simulink model "gnc"  (R2025b)
settings: Solver=ode2  StartTime=0.0  StopTime=inf  FixedStep=1/100  RelTol=1e-3
PreLoadFcn:
  | gnc_PreLoadFcn
undefined symbols (not defined in the file or in its folder): DiscIntNeverNeededParam, dspblkCoreblockFVToolHelper, gcbh
libraries: simulink_extras x7, simulink x5, eeGeneralControl x5
(part 3 of 4)

== system gnc/Subsystem2/Actuator_Model/Actuator Model ==
  note: Discrete time actuator
      | dynamics transfer function
      | modelled as PT1 in
      | continuous time (tau = 0.05,
      | ts = 100Hz).
      | See filter_design.m for
      | more details.
  note: Actuator model output units need to
      | match increment units of control law.
      | Therefore, controller output must be
      | retransformed to corresponding unit.
  note: Current control surface
      | deflection in rad, thrust
      | lever in [0,1].
  note: Current actuator signal in %
      | Thrust [-1, 1]
      | Aileron [-1, 1]
      | Elevator [-1, 1]
      | Rudder [-1, 1]
  note: Scale actuator
      | signal from
      | % to rad
  note: Limit between
      | [-1,1]
  note: Limit
      | between
      | [0,1]
  note: Discrete time thrust
      | dynamics transfer function
      | modelled as PT1 in
      | continuous time (tau = 0.15,
      | ts = 100Hz).
      | See filter_design.m for
      | more details.
  note: Aileron		[-1, 1]
      | Elevator		[-1, 1]
      | Rudder		[-1, 1]
      | Thrust		[0, 1]
  note: Scale thrust signal
  RC_controls : Inport
  Safety_Switch : Inport  Port=2
  AP_controls : Inport  Port=3  OutDataTypeStr=Bus: main_ctrl_axes_bus
  act_lims : Inport  Port=4
  Bus Selector : BusSelector  OutputSignals=aileron,elevator,rudder,thrust
  Data Type Conversion1 : DataTypeConversion  OutDataTypeStr=single  SaturateOnIntegerOverflow=off  RndMeth=Floor
  Demux : Demux
  MATLAB Function1 : MATLAB Function  TreatAsAtomicUnit=on
  Mux : Mux  Inputs=3
  Mux1 : Mux  Inputs=2
  Mux4 : Mux
  Scope : Scope  NumInputPorts=4
  Scope1 : Scope  NumInputPorts=4
      settings: ActiveDisplayYMinimum=-0.125  ActiveDisplayYMaximum=1.125
  Scope2 : Scope
      settings: ActiveDisplayYMinimum=-1  ActiveDisplayYMaximum=1  DataLoggingVariableName=ScopeData8
  Switch1 : Switch  Criteria=u2 > Threshold  SaturateOnIntegerOverflow=off  InputSameDT=off
  act_alg : DiscreteTransferFcn  Numerator=[0.0909 0.0909]  Denominator=[1 -0.8182]
  act_alg2 : DiscreteTransferFcn  LoadFcn=dspblkCoreblockFVToolHelper(gcbh,'load');  Numerator=[0.0323 0.0323]  Denominator=[1 -0.9355]
      settings: CopyFcn=dspblkCoreblockFVToolHelper(gcbh,'copy');  DeleteFcn=dspblkCoreblockFVToolHelper(gcbh,'close');  ModelCloseFcn=dspblkCoreblockFVToolHelper(gcbh,'close');  PreSaveFcn=dspblkCoreblockFVToolHelper(gcbh,'presave');  PostSaveFcn=dspblkCoreblockFVToolHelper(gcbh,'postsave');  CloseFcn=dspblkCoreblockFVToolHelper(gcbh,'close');
  cmd2deg : MATLAB Function  TreatAsAtomicUnit=on
  limit control output : MATLAB Function  TreatAsAtomicUnit=on
  limit control output3 : MATLAB Function  TreatAsAtomicUnit=on
  Delayed : Outport
  wires:
  act_alg2/1 -> Scope1/1, Mux1/2
  limit control output3/1(y) -> Scope1/2, act_alg2/1, Scope1/3
  act_lims/1 -> cmd2deg/1(act_limits)
  Mux1/1 -> Data Type Conversion1/1
  act_alg/1 -> Scope/4, Mux1/1
  Demux/3 -> Mux/3
  Demux/1 -> Mux/1
  Demux/2 -> Mux/2
  AP_controls/1 -> Bus Selector/1
  Data Type Conversion1/1 -> Delayed/1
  Mux4/1 -> MATLAB Function1/1(in), Scope2/1
  Mux/1 -> Scope/1, limit control output/1(u)
  cmd2deg/1(y) -> Scope/3, act_alg/1
  limit control output/1(y) -> Scope/2, cmd2deg/2(u)
  MATLAB Function1/1(out) -> Switch1/3
  Bus Selector/4 -> Mux4/4  "<thrust>"
  Demux/4 -> Scope1/4, limit control output3/1(u)
  RC_controls/1 -> Switch1/1
  Safety_Switch/1 -> Switch1/2
  Switch1/1 -> Demux/1
  Bus Selector/1 -> Mux4/1  "<aileron>"
  Bus Selector/2 -> Mux4/2  "<elevator>"
  Bus Selector/3 -> Mux4/3  "<rudder>"

== system gnc/Subsystem2/Actuator_Model/Subsystem1 ==
  note: Input from Gram RC:
      | 1 Thrust
      | 2 Aileron
      | 3 Elevator
      | 4 Rudder
      | 5 Tail surface right
      | 6 Tail surface left
      | 7 Mode switch
      | 8 Arming
      | 9 Safety
  note: (1) test_controls
      | (2) steady_state
      | (3) wp_tracking
  note: Signal Limits:
      | Aileron		[-1, 1]
      | Elevator		[-1, 1]
      | Rudder		[-1, 1]
      | Thrust		[0, 1]
  note: [ Aileron	  ]
      | [ Elevator ]
      | [ Rudder	  ]
      | [ Thrust	  ]
  RC_channels : Inport  OutDataTypeStr=Bus: rc_channels_bus
  Bus Selector1 : BusSelector  OutputSignals=channels
  Demux1 : Demux  Outputs=6
  MATLAB Function : MATLAB Function  TreatAsAtomicUnit=on
  Mux : Mux
  Scope : Scope  NumInputPorts=2
      settings: ActiveDisplayYMinimum=-1.5  ActiveDisplayYMaximum=3.5  DataLoggingVariableName=ScopeData3
  Scope1 : Scope
      settings: ActiveDisplayYMinimum=-1.5  ActiveDisplayYMaximum=3.5  DataLoggingVariableName=ScopeData7
  Selector : Selector  InputPortWidth=18  IndexOptions=Index vector (dialog)  Indices=[2 3 4 1 7 9]  OutputSizes=1
  rc_mode : Outport  OutDataTypeStr=uint8
  RC_controls : Outport  Port=2
  Safety_Switch : Outport  Port=3
  wires:
  Demux1/3 -> Mux/3
  Demux1/1 -> Mux/1
  Demux1/2 -> Mux/2
  MATLAB Function/1(y) -> Scope/1, rc_mode/1
  Selector/1 -> Demux1/1
  Mux/1 -> RC_controls/1
  Demux1/5 -> MATLAB Function/1(u), Scope/2
  RC_channels/1 -> Bus Selector1/1
  Demux1/6 -> Safety_Switch/1, Scope1/1
  Demux1/4 -> Mux/4
  Bus Selector1/1 -> Selector/1  "<channels>"

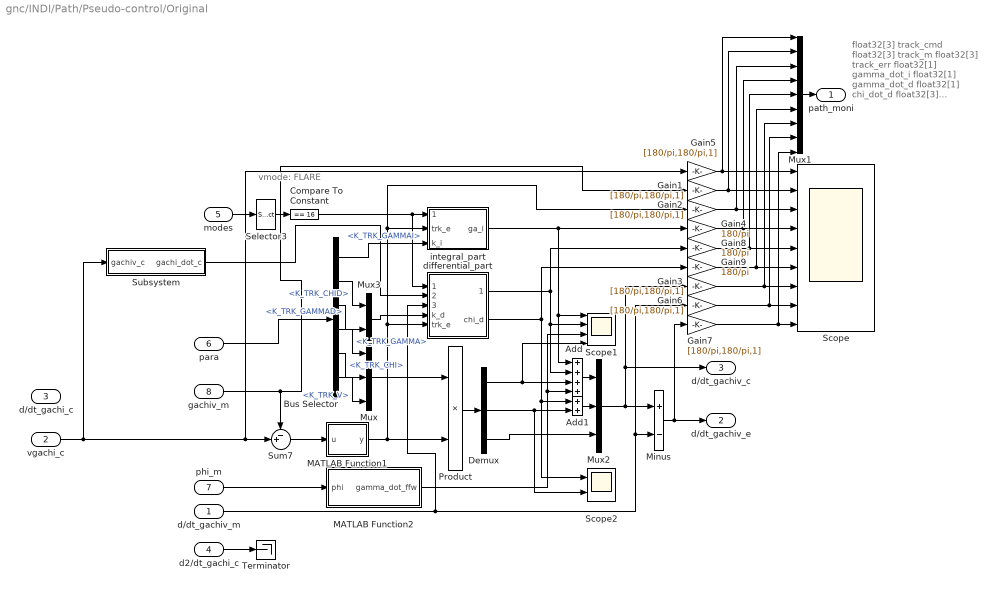
== system gnc/INDI/Path/Pseudo-control/Original ==
  note: float32[3] track_cmd
      | float32[3] track_m
      | float32[3] track_err
      | float32[1] gamma_dot_i
      | float32[1] gamma_dot_d
      | float32[1] chi_dot_d
      | float32[3] track_dot_cmd
      | float32[3] track_dot_m
      | float32[3] track_dot_err
  note: vmode: FLARE
  d/dt_gachiv_m : Inport  PortDimensions=3
  vgachi_c : Inport  Port=2
  d/dt_gachi_c : Inport  Port=3
  d2/dt_gachi_c : Inport  Port=4
  modes : Inport  Port=5  PortDimensions=4
  para : Inport  Port=6  OutDataTypeStr=Bus: gnc_parameterBus
  phi_m : Inport  Port=7
  gachiv_m : Inport  Port=8  PortDimensions=3
  Add : Sum  Inputs=++++
  Add1 : Sum
  Bus Selector : BusSelector  OutputSignals=indi.K_TRK_GAMMAI,indi.K_TRK_CHID,indi.K_TRK_GAMMAD,indi.K_TRK_GAMMA,indi.K_TRK_CHI,indi.K_TRK_V
  Compare To Constant : simulink/Logic and Bit Operations/Compare To Constant  relop===  const=16  OutDataTypeStr=boolean
  Demux : Demux  Outputs=3
  Gain{1..3,5..7} (6 alike) : Gain  Gain=[180/pi,180/pi,1]
  Gain4 : Gain  Gain=180/pi
  Gain8 : Gain  Gain=180/pi
  Gain9 : Gain  Gain=180/pi
  MATLAB Function1 : MATLAB Function  TreatAsAtomicUnit=on
  MATLAB Function2 : MATLAB Function  TreatAsAtomicUnit=on
  Minus : Sum  Inputs=+-
  Mux : Mux  Inputs=3
  Mux1 : Mux  Inputs=9
  Mux2 : Mux  Inputs=3
  Mux3 : Mux  Inputs=2
  Product : Product
  Scope : Scope  NumInputPorts=9
      settings: ActiveDisplayYMinimum=-85.31239  ActiveDisplayYMaximum=124.63703
  Scope1 : Scope  NumInputPorts=4
      settings: ActiveDisplayYMinimum=-1  ActiveDisplayYMaximum=1  DataLoggingVariableName=ScopeData2
  Scope2 : Scope  NumInputPorts=2
      settings: ActiveDisplayYMinimum=-1  ActiveDisplayYMaximum=1  DataLoggingVariableName=ScopeData2
  Selector3 : Selector  InputPortWidth=4  IndexOptions=Index vector (dialog)  Indices=1  OutputSizes=1
  Subsystem : Subsystem
  Sum7 : Sum  Inputs=-+|
  Terminator : Terminator
  differential_part : Subsystem
  integral_part : Subsystem
  path_moni : Outport
  d/dt_gachiv_e : Outport  Port=2  OutDataTypeStr=single  PortDimensions=3
  d/dt_gachiv_c : Outport  Port=3  OutDataTypeStr=single  PortDimensions=3
  wires:
  Gain6/1 -> Mux1/8, Scope/8
  vgachi_c/1 -> Subsystem/1(gachiv_c), Gain5/1, Sum7/2
  Minus/1 -> d/dt_gachiv_e/1, Gain7/1
  Gain4/1 -> Mux1/4, Scope/4
  Subsystem/1(gachi_dot_c) -> differential_part/2(gachi_dot_c)
  Gain9/1 -> Mux1/6, Scope/6
  Demux/1 -> Scope1/4, Add/3
  phi_m/1 -> MATLAB Function2/1(phi)
  Product/1 -> Demux/1
  Add1/1 -> Mux2/2
  Mux3/1 -> differential_part/4(k_d)
  Gain5/1 -> Mux1/1, Scope/1
  Gain7/1 -> Mux1/9, Scope/9
  Bus Selector/2 -> Mux3/1  "<K_TRK_CHID>"
  Sum7/1 -> MATLAB Function1/1(u)
  Compare To Constant/1 -> differential_part/1(flare_trig), integral_part/1(flare_trig)
  d/dt_gachiv_m/1 -> differential_part/3(gachiv_dot_m), Gain6/1, Minus/2
  Demux/3 -> Mux2/3
  Mux1/1 -> path_moni/1
  MATLAB Function2/1(gamma_dot_ffw) -> Add/4, Scope1/3
  Bus Selector/1 -> integral_part/3(k_i)  "<K_TRK_GAMMAI>"
  integral_part/1(ga_i) -> Add/1, Scope1/1, Gain4/1
  differential_part/1(gamma_d) -> Gain8/1, Add/2, Scope1/2
  Gain8/1 -> Mux1/5, Scope/5
  Mux/1 -> Product/1
  differential_part/2(chi_d) -> Gain9/1, Scope2/1, Add1/1
  Gain3/1 -> Mux1/7, Scope/7
  modes/1 -> Selector3/1
  Bus Selector/5 -> Mux/2  "<K_TRK_CHI>"
  d2/dt_gachi_c/1 -> Terminator/1
  Bus Selector/4 -> Mux/1  "<K_TRK_GAMMA>"
  Gain1/1 -> Mux1/2, Scope/2
  gachiv_m/1 -> Sum7/1, Gain1/1
  Mux2/1 -> Minus/1, d/dt_gachiv_c/1, Gain3/1
  Bus Selector/6 -> Mux/3  "<K_TRK_V>"
  MATLAB Function1/1(y) -> differential_part/5(trk_e), Gain2/1, integral_part/2(trk_e), Product/2
  Add/1 -> Mux2/1
  para/1 -> Bus Selector/1
  Bus Selector/3 -> Mux3/2  "<K_TRK_GAMMAD>"
  Gain2/1 -> Mux1/3, Scope/3
  Demux/2 -> Scope2/2, Add1/2
  Selector3/1 -> Compare To Constant/1

== system gnc/INDI/Path/Pseudo-control/wrap2Pi ==
  note: Wrap input to [-pi,pi)
  In1 : Inport  OutDataTypeStr=single
  Add : Sum
  Constant3 : Constant  Value=single(pi)  OutDataTypeStr=single
  Gain : Gain  Gain=2
  Subtract1 : Sum  Inputs=+-
  mathFunction : Math  Operator=mod  SignedPower=on
  Out1 : Outport  OutDataTypeStr=single
  wires:
  mathFunction/1 -> Subtract1/1
  Gain/1 -> mathFunction/2
  Subtract1/1 -> Out1/1
  In1/1 -> Add/1
  Add/1 -> mathFunction/1
  Constant3/1 -> Subtract1/2, Gain/1, Add/2

== system gnc/INDI/Rates to surfaces&brakes/Diff and Filter IMU/Subsystem ==
  note: Discrete time IMU derivative and
      | second order washout filter transfer function
      | (omega = 90, zeta = 1, ts = 100Hz).
      | See filter_design.m for more details.
  note: Discrete time second order washout filter
      | (omega = 90, zeta = 1, ts = 100Hz) transfer
      | function to synchronize phase shift between
      | IMU derivative and actuator position signals.
      | See filter_design.m for more details.
  rates : Inport
  act_m : Inport  Port=2
  Scope : Scope  NumInputPorts=2
  Scope1 : Scope  NumInputPorts=2
  imu_alg : DiscreteTransferFcn  Numerator=[0.0963 0.1926 0.0963]  Denominator="[1 -0.7586  0.1439]"
  imu_dt_alg : DiscreteTransferFcn  Numerator=[19.2628 0 -19.2628]  Denominator=[1 -0.7586 0.1439]
  dt_pqr_m : Outport
  act_del : Outport  Port=2
  wires:
  imu_dt_alg/1 -> dt_pqr_m/1, Scope1/2
  rates/1 -> Scope1/1, imu_dt_alg/1
  imu_alg/1 -> act_del/1, Scope/1
  act_m/1 -> Scope/2, imu_alg/1

== system gnc/INDI/Rates to surfaces&brakes/Diff and Filter IMU/fromRPAS ==
  note: Filter eigenfrequency in rad/s
  note: Discrete time IMU derivative and
      | second order washout filter transfer function.
      | See filter_design.m for more details.
  note: Discrete time second order washout filter
      | to synchronize phase shift between
      | IMU derivative and actuator position signals.
      | See filter_design.m for more details.
  note: Filter damping
  act_m : Inport
  rates : Inport  Port=2
  Constant : Constant  Value=20  OutDataTypeStr=single
  Constant1 : Constant  OutDataTypeStr=single
  Discrete Transfer Fcn1 : DiscreteTransferFcn  NumeratorSource=Input port  DenominatorSource=Input port  a0EqualsOne=on
      settings: InputPortMap=u0,p1,p3
  Discrete Transfer Fcn2 : DiscreteTransferFcn  NumeratorSource=Input port  DenominatorSource=Input port  a0EqualsOne=on
      settings: InputPortMap=u0,p1,p3
  Discrete Transfer Fcn3 : DiscreteTransferFcn  NumeratorSource=Input port  DenominatorSource=Input port  a0EqualsOne=on
      settings: InputPortMap=u0,p1,p3
  Display{,1..3} (4 alike) : Display
  MATLAB Function : MATLAB Function  TreatAsAtomicUnit=on
  Scope : Scope  NumInputPorts=2
  Selector : Selector  InputPortWidth=4  IndexOptions=Index vector (dialog)  Indices=1:3  OutputSizes=1
  Subsystem : Subsystem
  Transpose{,1..3} (4 alike) : Math  Operator=transpose
  act_del : Outport  OutDataTypeStr=single  PortDimensions=3
  d/dt_pqr_m : Outport  Port=2  OutDataTypeStr=single  PortDimensions=3
  wires:
  act_m/1 -> Selector/1
  Selector/1 -> Discrete Transfer Fcn2/1
  rates/1 -> Discrete Transfer Fcn3/1, Subsystem/1(In1), Scope/1, Discrete Transfer Fcn1/1
  MATLAB Function/1(diff_num) -> Transpose/1, Discrete Transfer Fcn1/2
  MATLAB Function/2(diff_den) -> Transpose1/1, Discrete Transfer Fcn1/3
  MATLAB Function/3(filt_num) -> Transpose2/1, Discrete Transfer Fcn3/2, Discrete Transfer Fcn2/2
  MATLAB Function/4(filt_den) -> Transpose3/1, Discrete Transfer Fcn3/3, Discrete Transfer Fcn2/3
  Constant/1 -> MATLAB Function/1(omega)
  Constant1/1 -> MATLAB Function/2(zeta)
  Discrete Transfer Fcn2/1 -> act_del/1
  Discrete Transfer Fcn1/1 -> d/dt_pqr_m/1
  Transpose/1 -> Display/1
  Transpose1/1 -> Display1/1
  Transpose2/1 -> Display2/1
  Transpose3/1 -> Display3/1
  Discrete Transfer Fcn3/1 -> Scope/2

== system gnc/INDI/Path/Pseudo-control/Original/Subsystem ==
  note: Discrete time IMU derivative and
      | second order washout filter transfer function
      | (omega = 90, zeta = 1, ts = 100Hz).
      | See filter_design.m for more details.
  gachiv_c : Inport  OutDataTypeStr=single  PortDimensions=3
  Scope : Scope  NumInputPorts=2
      settings: ActiveDisplayYMinimum=-3.92699  ActiveDisplayYMaximum=3.92699  DataLoggingVariableName=ScopeData6
  Selector : Selector  InputPortWidth=3  IndexOptions=Index vector (dialog)  Indices=1:2  OutputSizes=1
  imu_dt_alg : DiscreteTransferFcn  Numerator=[19.2628 0 -19.2628]  Denominator=[1 -0.7586 0.1439]
  gachi_dot_c : Outport  OutDataTypeStr=single  PortDimensions=2
  wires:
  gachiv_c/1 -> Selector/1
  imu_dt_alg/1 -> Scope/2, gachi_dot_c/1
  Selector/1 -> Scope/1, imu_dt_alg/1

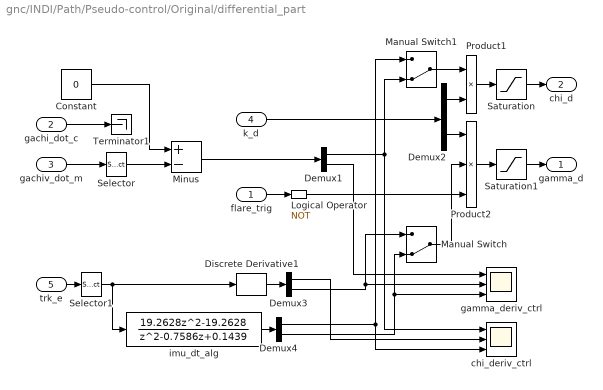
== system gnc/INDI/Path/Pseudo-control/Original/differential_part ==
  flare_trig : Inport
  gachi_dot_c : Inport  Port=2  OutDataTypeStr=single  PortDimensions=2
  gachiv_dot_m : Inport  Port=3
  k_d : Inport  Port=4
  trk_e : Inport  Port=5
  Constant : Constant  Value=0  OutDataTypeStr=single
  Demux{1..4} (4 alike) : Demux  Outputs=2
  Discrete Derivative1 : simulink/Discrete/Discrete Derivative  gainval=1.0  ICPrevScaledInput=0.0  OutMin=[]  OutMax=[]  OutDataType=fixdt(1, 16)  OutScaling=2^-10  DoSatur=off
  Logical Operator : Logic  Operator=NOT  AllPortsSameDT=off  OutDataTypeStr=boolean
  Manual Switch : ManualSwitch  CurrentSetting=0
  Manual Switch1 : ManualSwitch  CurrentSetting=0
  Minus : Sum  Inputs=+-
  Product1 : Product
  Product2 : Product  Inputs=3
  Saturation : Saturate  UpperLimit=1  LowerLimit=-1  OutDataTypeStr=single
  Saturation1 : Saturate  UpperLimit=1  LowerLimit=-1  OutDataTypeStr=single
  Selector : Selector  InputPortWidth=3  IndexOptions=Index vector (dialog)  Indices=[2,1]  OutputSizes=1
  Selector1 : Selector  InputPortWidth=3  IndexOptions=Index vector (dialog)  Indices=[2,1]  OutputSizes=1
  Terminator1 : Terminator
  chi_deriv_ctrl : Scope  NumInputPorts=3
  gamma_deriv_ctrl : Scope  NumInputPorts=3
  imu_dt_alg : DiscreteTransferFcn  Numerator=[19.2628 0 -19.2628]  Denominator=[1 -0.7586 0.1439]
  gamma_d : Outport
  chi_d : Outport  Port=2
  wires:
  Demux1/2 -> gamma_deriv_ctrl/1
  Demux3/1 -> chi_deriv_ctrl/2
  trk_e/1 -> Selector1/1
  Discrete Derivative1/1 -> Demux3/1
  Selector1/1 -> Discrete Derivative1/1, imu_dt_alg/1
  k_d/1 -> Demux2/1
  Minus/1 -> Demux1/1
  flare_trig/1 -> Logical Operator/1
  Selector/1 -> Minus/2
  gachiv_dot_m/1 -> Selector/1
  Logical Operator/1 -> Product2/3
  Product1/1 -> Saturation/1
  Demux1/1 -> chi_deriv_ctrl/1, Manual Switch1/2
  Demux2/1 -> Product1/2
  Demux2/2 -> Product2/1
  gachi_dot_c/1 -> Terminator1/1
  Product2/1 -> Saturation1/1
  Demux3/2 -> gamma_deriv_ctrl/2, Manual Switch/1
  Constant/1 -> Minus/1
  Manual Switch/1 -> Product2/2
  Demux4/2 -> gamma_deriv_ctrl/3, Manual Switch/2
  imu_dt_alg/1 -> Demux4/1
  Demux4/1 -> chi_deriv_ctrl/3, Manual Switch1/1
  Manual Switch1/1 -> Product1/1
  Saturation/1 -> chi_d/1
  Saturation1/1 -> gamma_d/1

== system gnc/INDI/Path/Pseudo-control/Original/integral_part ==
  flare_trig : Inport
  trk_e : Inport  Port=2
  k_i : Inport  Port=3
  Discrete-Time Integrator : DiscreteIntegrator  ExternalReset=rising  SampleTime=-1  LimitOutput=on  UpperSaturationLimit=1  LowerSaturationLimit=-1  ICPrevOutput=DiscIntNeverNeededParam  ICPrevScaledInput=DiscIntNeverNeededParam
  Gain4 : Gain  Gain=0
  Product2 : Product  Inputs=3
  Selector : Selector  InputPortWidth=3  IndexOptions=Index vector (dialog)  Indices=1  OutputSizes=1
  ga_i : Outport
  wires:
  trk_e/1 -> Selector/1
  Selector/1 -> Discrete-Time Integrator/1
  flare_trig/1 -> Discrete-Time Integrator/2, Product2/2
  Product2/1 -> Gain4/1
  Gain4/1 -> ga_i/1
  Discrete-Time Integrator/1 -> Product2/1
  k_i/1 -> Product2/3

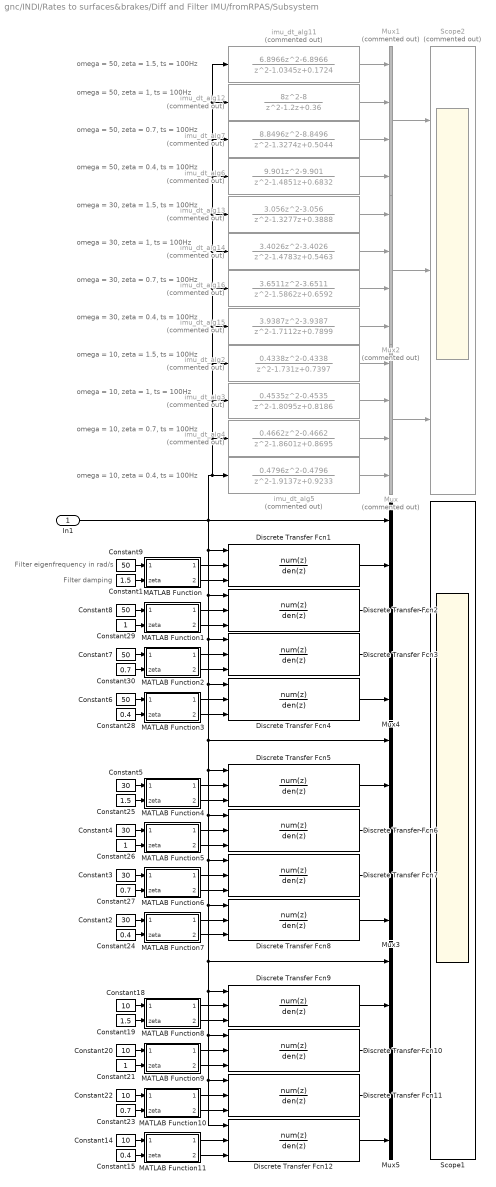
== system gnc/INDI/Rates to surfaces&brakes/Diff and Filter IMU/fromRPAS/Subsystem ==
  note: omega = 10, zeta = 1.5, ts = 100Hz
  note: omega = 10, zeta = 1, ts = 100Hz
  note: omega = 10, zeta = 0.7, ts = 100Hz
  note: omega = 10, zeta = 0.4, ts = 100Hz
  note: omega = 50, zeta = 0.4, ts = 100Hz
  note: omega = 30, zeta = 0.4, ts = 100Hz
  note: omega = 50, zeta = 1.5, ts = 100Hz
  note: omega = 50, zeta = 1, ts = 100Hz
  note: omega = 50, zeta = 0.7, ts = 100Hz
  note: omega = 30, zeta = 0.7, ts = 100Hz
  note: omega = 30, zeta = 1.5, ts = 100Hz
  note: omega = 30, zeta = 1, ts = 100Hz
  note: Filter eigenfrequency in rad/s
  note: Filter damping
  In1 : Inport
  Constant1 : Constant  Value=1.5  OutDataTypeStr=single
  Constant{14,18,20,22} (4 alike) : Constant  Value=10  OutDataTypeStr=single
  Constant15 : Constant  Value=0.4  OutDataTypeStr=single
  Constant19 : Constant  Value=1.5  OutDataTypeStr=single
  Constant{2..5} (4 alike) : Constant  Value=30  OutDataTypeStr=single
  Constant21 : Constant  OutDataTypeStr=single
  Constant23 : Constant  Value=0.7  OutDataTypeStr=single
  Constant24 : Constant  Value=0.4  OutDataTypeStr=single
  Constant25 : Constant  Value=1.5  OutDataTypeStr=single
  Constant26 : Constant  OutDataTypeStr=single
  Constant27 : Constant  Value=0.7  OutDataTypeStr=single
  Constant28 : Constant  Value=0.4  OutDataTypeStr=single
  Constant29 : Constant  OutDataTypeStr=single
  Constant30 : Constant  Value=0.7  OutDataTypeStr=single
  Constant{6..9} (4 alike) : Constant  Value=50  OutDataTypeStr=single
  Discrete Transfer Fcn{1..12} (12 alike) : DiscreteTransferFcn  NumeratorSource=Input port  DenominatorSource=Input port  a0EqualsOne=on
      settings: InputPortMap=u0,p1,p3
  MATLAB Function : MATLAB Function  TreatAsAtomicUnit=on
  MATLAB Function1 : MATLAB Function  TreatAsAtomicUnit=on
  MATLAB Function10 : MATLAB Function  TreatAsAtomicUnit=on
  MATLAB Function11 : MATLAB Function  TreatAsAtomicUnit=on
  MATLAB Function2 : MATLAB Function  TreatAsAtomicUnit=on
  MATLAB Function3 : MATLAB Function  TreatAsAtomicUnit=on
  MATLAB Function4 : MATLAB Function  TreatAsAtomicUnit=on
  MATLAB Function5 : MATLAB Function  TreatAsAtomicUnit=on
  MATLAB Function6 : MATLAB Function  TreatAsAtomicUnit=on
  MATLAB Function7 : MATLAB Function  TreatAsAtomicUnit=on
  MATLAB Function8 : MATLAB Function  TreatAsAtomicUnit=on
  MATLAB Function9 : MATLAB Function  TreatAsAtomicUnit=on
  Mux : Mux  Commented=on
  Mux1 : Mux  Commented=on
  Mux2 : Mux  Commented=on
  Mux3 : Mux  Inputs=5
  Mux4 : Mux  Inputs=5
  Mux5 : Mux  Inputs=5
  Scope1 : Scope  NumInputPorts=3
      settings: ActiveDisplayYMinimum=-0.91267  ActiveDisplayYMaximum=1.00595
  Scope2 : Scope  Commented=on  NumInputPorts=3
      settings: ActiveDisplayYMinimum=-0.91267  ActiveDisplayYMaximum=1.00595
  imu_dt_alg11 : DiscreteTransferFcn  Commented=on  Numerator=[6.8966 0 -6.8966]  Denominator=[1 -1.0345 0.1724]
  imu_dt_alg12 : DiscreteTransferFcn  Commented=on  Numerator=[8 0 -8]  Denominator=[1 -1.2 0.36]
  imu_dt_alg13 : DiscreteTransferFcn  Commented=on  Numerator=[3.056 0 -3.056]  Denominator=[1 -1.3277 0.3888]
  imu_dt_alg14 : DiscreteTransferFcn  Commented=on  Numerator=[3.4026 0 -3.4026]  Denominator=[1 -1.4783 0.5463]
  imu_dt_alg15 : DiscreteTransferFcn  Commented=on  Numerator=[3.9387 0 -3.9387]  Denominator=[1 -1.7112 0.7899]
  imu_dt_alg16 : DiscreteTransferFcn  Commented=on  Numerator=[3.6511 0 -3.6511]  Denominator=[1 -1.5862 0.6592]
  imu_dt_alg2 : DiscreteTransferFcn  Commented=on  Numerator=[0.4338 0 -0.4338]  Denominator=[1 -1.731 0.7397]
  imu_dt_alg3 : DiscreteTransferFcn  Commented=on  Numerator=[0.4535 0 -0.4535]  Denominator=[1 -1.8095 0.8186]
  imu_dt_alg4 : DiscreteTransferFcn  Commented=on  Numerator=[0.4662 0 -0.4662]  Denominator=[1 -1.8601 0.8695]
  imu_dt_alg5 : DiscreteTransferFcn  Commented=on  Numerator=[0.4796 0 -0.4796]  Denominator=[1 -1.9137 0.9233]
  imu_dt_alg6 : DiscreteTransferFcn  Commented=on  Numerator=[9.901 0 -9.901]  Denominator=[1 -1.4851 0.6832]
  imu_dt_alg7 : DiscreteTransferFcn  Commented=on  Numerator=[8.8496 0 -8.8496]  Denominator=[1 -1.3274 0.5044]
  wires:
  imu_dt_alg4/1 -> Mux/3
  imu_dt_alg3/1 -> Mux/2
  imu_dt_alg6/1 -> Mux1/4
  imu_dt_alg5/1 -> Mux/4
  imu_dt_alg13/1 -> Mux2/1
  imu_dt_alg7/1 -> Mux1/3
  imu_dt_alg2/1 -> Mux/1
  imu_dt_alg11/1 -> Mux1/1
  Mux1/1 -> Scope2/1
  imu_dt_alg16/1 -> Mux2/3
  imu_dt_alg15/1 -> Mux2/4
  imu_dt_alg14/1 -> Mux2/2
  imu_dt_alg12/1 -> Mux1/2
  Mux/1 -> Scope2/3
  Mux2/1 -> Scope2/2
  Constant1/1 -> MATLAB Function/2(zeta)
  Constant9/1 -> MATLAB Function/1(omega)
  MATLAB Function/1(filt_num) -> Discrete Transfer Fcn1/2
  MATLAB Function/2(filt_den) -> Discrete Transfer Fcn1/3
  Constant8/1 -> MATLAB Function1/1(omega)
  Constant29/1 -> MATLAB Function1/2(zeta)
  Constant30/1 -> MATLAB Function2/2(zeta)
  Constant7/1 -> MATLAB Function2/1(omega)
  Constant28/1 -> MATLAB Function3/2(zeta)
  Constant25/1 -> MATLAB Function4/2(zeta)
  Constant5/1 -> MATLAB Function4/1(omega)
  Constant4/1 -> MATLAB Function5/1(omega)
  Constant26/1 -> MATLAB Function5/2(zeta)
  Constant15/1 -> MATLAB Function11/2(zeta)
  Constant14/1 -> MATLAB Function11/1(omega)
  Constant22/1 -> MATLAB Function10/1(omega)
  Constant23/1 -> MATLAB Function10/2(zeta)
  Constant21/1 -> MATLAB Function9/2(zeta)
  Constant20/1 -> MATLAB Function9/1(omega)
  Constant18/1 -> MATLAB Function8/1(omega)
  Constant19/1 -> MATLAB Function8/2(zeta)
  Constant24/1 -> MATLAB Function7/2(zeta)
  Constant2/1 -> MATLAB Function7/1(omega)
  Constant3/1 -> MATLAB Function6/1(omega)
  Constant27/1 -> MATLAB Function6/2(zeta)
  MATLAB Function11/2(filt_den) -> Discrete Transfer Fcn12/3
  MATLAB Function11/1(filt_num) -> Discrete Transfer Fcn12/2
  MATLAB Function10/2(filt_den) -> Discrete Transfer Fcn11/3
  MATLAB Function10/1(filt_num) -> Discrete Transfer Fcn11/2
  MATLAB Function9/2(filt_den) -> Discrete Transfer Fcn10/3
  MATLAB Function9/1(filt_num) -> Discrete Transfer Fcn10/2
  MATLAB Function8/2(filt_den) -> Discrete Transfer Fcn9/3
  MATLAB Function8/1(filt_num) -> Discrete Transfer Fcn9/2
  MATLAB Function7/2(filt_den) -> Discrete Transfer Fcn8/3
  MATLAB Function7/1(filt_num) -> Discrete Transfer Fcn8/2
  MATLAB Function6/2(filt_den) -> Discrete Transfer Fcn7/3
  MATLAB Function6/1(filt_num) -> Discrete Transfer Fcn7/2
  In1/1 -> imu_dt_alg14/1, imu_dt_alg13/1, imu_dt_alg6/1, imu_dt_alg7/1, imu_dt_alg12/1, imu_dt_alg11/1, imu_dt_alg16/1, imu_dt_alg15/1, imu_dt_alg2/1, imu_dt_alg3/1, imu_dt_alg4/1, imu_dt_alg5/1, Mux3/1, Discrete Transfer Fcn5/1, Discrete Transfer Fcn12/1, Discrete Transfer Fcn11/1, Discrete Transfer Fcn10/1, Discrete Transfer Fcn9/1, Mux5/1, Discrete Transfer Fcn8/1, Discrete Transfer Fcn7/1, Discrete Transfer Fcn6/1, Discrete Transfer Fcn4/1, Discrete Transfer Fcn3/1, Discrete Transfer Fcn2/1, Discrete Transfer Fcn1/1, Mux4/1
  MATLAB Function5/2(filt_den) -> Discrete Transfer Fcn6/3
  MATLAB Function5/1(filt_num) -> Discrete Transfer Fcn6/2
  MATLAB Function4/2(filt_den) -> Discrete Transfer Fcn5/3
  MATLAB Function4/1(filt_num) -> Discrete Transfer Fcn5/2
  MATLAB Function3/2(filt_den) -> Discrete Transfer Fcn4/3
  MATLAB Function3/1(filt_num) -> Discrete Transfer Fcn4/2
  MATLAB Function2/2(filt_den) -> Discrete Transfer Fcn3/3
  MATLAB Function2/1(filt_num) -> Discrete Transfer Fcn3/2
  MATLAB Function1/2(filt_den) -> Discrete Transfer Fcn2/3
  MATLAB Function1/1(filt_num) -> Discrete Transfer Fcn2/2
  Constant6/1 -> MATLAB Function3/1(omega)
  Mux3/1 -> Scope1/2
  Mux5/1 -> Scope1/3
  Mux4/1 -> Scope1/1
  Discrete Transfer Fcn1/1 -> Mux4/2
  Discrete Transfer Fcn2/1 -> Mux4/3
  Discrete Transfer Fcn3/1 -> Mux4/4
  Discrete Transfer Fcn4/1 -> Mux4/5
  Discrete Transfer Fcn5/1 -> Mux3/2
  Discrete Transfer Fcn6/1 -> Mux3/3
  Discrete Transfer Fcn7/1 -> Mux3/4
  Discrete Transfer Fcn8/1 -> Mux3/5
  Discrete Transfer Fcn9/1 -> Mux5/2
  Discrete Transfer Fcn10/1 -> Mux5/3
  Discrete Transfer Fcn11/1 -> Mux5/4
  Discrete Transfer Fcn12/1 -> Mux5/5

== matlab function gnc/INDI/limit control output ==
  data: u input; y output single
function y = control_output_sat(u)
%outputs scaled according to API definition
limit = 1;

y = u;
y(1:3) = min(max(u(1:3),-limit),limit);
y(4)   = min(max(u(4),0),limit);
end

== matlab function gnc/lla2ned ==
  settings: updateMethod=DISCRETE
  data: lla0 input single size=3; WP_llu input Bus: waypoint_list_bus; wp_ned output single size=[3,20]; wp_count output size=1
function [wp_ned,wp_count]  = WPselector(lla0,WP_llu)

persistent waypoints_stored_lat waypoints_stored_lon waypoints_stored_alt waypoints_stored_count
NUM_WP = 20;

if (isempty(waypoints_stored_lat) || isempty(waypoints_stored_lon) || isempty(waypoints_stored_alt) || isempty(waypoints_stored_count))
    waypoints_stored_lat = zeros([NUM_WP,1], 'single');
    waypoints_stored_lon = zeros([NUM_WP,1], 'single');
    waypoints_stored_alt = zeros([NUM_WP,1], 'single');
    waypoints_stored_count = single(0);
end

llaRawToNed = single([0.011; 0.007; -0.001]);
lla_ref = single([487396608.0; 89221688.0; 483623.0]);

if (lla0)
    lla_ref = lla0;
    llaRawToNed = lla2ned(lla_ref);
end

% missionMonitor.is_valid = true;
% missionMonitor.wp_valid = double(WP_llu.is_valid);

if ((WP_llu.lat(1)) && (WP_llu.count)<NUM_WP+1 && (WP_llu.count)>0)
    waypoints_stored_lat = single(WP_llu.lat);
    waypoints_stored_lon = single(WP_llu.lon);
    waypoints_stored_alt = single(WP_llu.alt);
    waypoints_stored_count = single(WP_llu.count);
end

wp_north = zeros(NUM_WP,1,'single');
wp_east = zeros(NUM_WP,1,'single');
wp_down = zeros(NUM_WP,1,'single');
wp_count = single(0);
if (((waypoints_stored_count) > 0) && ((waypoints_stored_count) < NUM_WP+1))
    wp_count = waypoints_stored_count;
    for i=2:(waypoints_stored_count+1)
        coordsLlu = [waypoints_stored_lat(i-1)*1e7, waypoints_stored_lon(i-1)*1e7, waypoints_stored_alt(i-1)*1e3];
        coordsNED = llaRawToNed(1:2).*(coordsLlu(1:2)'-lla_ref(1:2));
        wp_north(i-1) = coordsNED(1);
        wp_east(i-1) = coordsNED(2);
        wp_down(i-1) = -waypoints_stored_alt(i-1);
    end
end
wp_ned = [wp_north';wp_east';wp_down'];
end

function llhRawToNed = lla2ned(llaRef)
semiMajorAxis=single(6378137);
eccentricity=single(8.1819190842622e-2);
posScaleFactor=single([1e-7*pi/180; 1e-7*pi/180; 1e-3]);
lattitudeRef=posScaleFactor(1)*single(llaRef(1)); %[rad]
heightRef=posScaleFactor(3)*single(llaRef(3)); %[m]
R0=semiMajorAxis/sqrt(1-eccentricity^2*sin(lattitudeRef)^2);
llhRawToNed=[(1-eccentricity^2)/semiMajorAxis^2*R0^3+heightRef; (R0+heightRef)*cos(lattitudeRef); -1].*posScaleFactor;
end

== matlab function gnc/Guidance/axisModes ==
  data: axis_modes output int8; AP_mode input uint8
function axis_modes  = fcn(AP_mode)

axis_modes = zeros(4,1,'int8'); %roll pitch yaw thrust
switch AP_mode
    case 1 %test_controls
        axis_modes(1) = int8(10); %AIL: PHI
        axis_modes(2) = int8(21); %ELE: THETA
        axis_modes(3) = int8(20); %RUD: PSI
        axis_modes(4) = int8(-1); %THR: IDLE
    case 2 %steady_state
        axis_modes(1) = int8(10); %AIL: PHI
        axis_modes(2) = int8(40); %ELE: GAMMA
        axis_modes(3) = int8(50); %RUD: SIDE_MIN
        axis_modes(4) = int8(10); %THR: SPD
    otherwise %flight path tracking
        axis_modes(1) = int8(40); %AIL: HDG
        axis_modes(2) = int8(40); %ELE: GAMMA
        axis_modes(3) = int8(50); %RUD: SIDE_MIN
        axis_modes(4) = int8(10); %THR: SPD
end

== matlab function gnc/INDI/MATLAB Function ==
  data: axis_modes input; thr_cmd output; thr input
function thr_cmd = fcn(axis_modes, thr)

if axis_modes(4) <= 0 %direct thrust
    thr_cmd = single(0);
else
    thr_cmd = thr;
end

== matlab function gnc/INDI/Attitude/Nonlinear_inversion/Limit_command ==
  data: param input; pqr_c input; rates_ltd output
function rates_ltd = fcn(param,pqr_c)

p_c = min(max(pqr_c(1),-param.limit.p_lim),param.limit.p_lim);
q_c = min(max(pqr_c(2),-param.limit.q_lim),param.limit.q_lim);
r_c  = min(max(pqr_c(3),-param.limit.r_lim),param.limit.r_lim);

rates_ltd = [p_c,q_c,r_c]';

== matlab function gnc/INDI/Attitude/MATLAB Function ==
  data: direct input; guidance input; modes input int8; att_c output
function att_c = fcn(direct,guidance,modes)

att_c = guidance;

if modes(1) == int8(10) %TEST_ROLL: PHI --> Xi
    att_c(5) = direct(5);
end

if modes(2) == int8(21) %VNAV_THETA: THETA --> ETA
    att_c(2) = direct(2);
end

if modes(3) == int8(20) %LNAV_ALGN: PSI --> ZETA
    att_c(4) = direct(4);
end

== matlab function gnc/Guidance/reset waypoints ==
  data: WP input; cruise_sw input uint8; reset output
function reset = resetWP(WP,cruise_sw)

persistent waypoints_old switch_old

if isempty(waypoints_old)
    waypoints_old = WP;
end
if isempty(switch_old)
    switch_old = cruise_sw;
end

reset = single(~isequal(WP, waypoints_old)||~isequal(cruise_sw, switch_old));

waypoints_old = WP;
switch_old = cruise_sw;

== matlab function gnc/INDI/Attitude/Nonlinear_inversion/Rate_Command_Generator ==
  data: att_dot_cmd input; gachiv_dot_m input single size=3; gamma_m input; modes input; att_m input; pqr_cmd output size=3
function pqr_cmd = tbv(att_dot_cmd,gachiv_dot_m,gamma_m,modes,att_m)
T_att = zeros(3,3,'single');
pseudo_angles = zeros(3,1,'single');

alpha = att_m(1);
theta = att_m(2);
beta  = att_m(3);
mu    = att_m(5);

T_bk = [cos(alpha)*cos(beta), sin(alpha)*sin(mu)-cos(alpha)*cos(mu)*sin(beta), -cos(mu)*sin(alpha)-cos(alpha)*sin(beta)*sin(mu);
    sin(beta), cos(beta)*cos(mu), cos(beta)*sin(mu);
    cos(beta)*sin(alpha), -cos(alpha)*sin(mu)-cos(mu)*sin(alpha)*sin(beta), cos(alpha)*cos(mu)-sin(alpha)*sin(beta)*sin(mu)];

T_alpha = [-cos(alpha)*tan(beta), 1, -sin(alpha)*tan(beta)];%alpha row: alpha_dot = T_alpha * (p q r)^T + path_vector(2)
T_theta = [0, cos(mu), -sin(mu)];%theta row: theta_dot = T_theta * (p q r)^T
T_beta = [sin(alpha), 0, -cos(alpha)];%beta row: beta_dot = T_beta * (p q r)^T + path_vector(3)
T_psi = [0, sin(mu)/cos(theta), cos(mu)/cos(theta)];%psi row: psi_dot = T_psi * (p q r)^T
T_mu = [cos(alpha)/cos(beta), 0 sin(alpha)/cos(beta)];%mu row: mu_dot = T_mu * (p q r)^T + path_vector(1)

% [alpha;beta;mu]_dot = Tatt*[p;q;r] - Tatt*T_bk*path_rotation = Tatt*[p,q,r] - path_vector
path_rot = [-gachiv_dot_m(2)*sin(gamma_m); gachiv_dot_m(1); gachiv_dot_m(2)*cos(gamma_m)];
path_vector = [T_alpha;T_beta;T_mu] * T_bk * path_rot;

if modes(2) == int8(21) %VNAV_THETA: THETA --> ETA
    T_att(1,:) = T_theta;
    pseudo_angles(1) = att_dot_cmd(2); %theta_dot_cmd
else
    T_att(1,:) = T_alpha;
    pseudo_angles(1) = att_dot_cmd(1)+path_vector(1); %alpha_dot_cmd + q_hat
end
if modes(3) == int8(20) %LNAV_ALGN: PSI --> ZETA
    T_att(2,:) = T_psi;
    pseudo_angles(2) = att_dot_cmd(4); %psi_dot_cmd
else
    T_att(2,:) = T_beta;
    pseudo_angles(2) = att_dot_cmd(3)+path_vector(2); %beta_dot_cmd + r_hat
end
T_att(3,:) = T_mu;
pseudo_angles(3) = att_dot_cmd(5)+path_vector(3); %mu_dot_cmd + p_hat

pqr_cmd = T_att\pseudo_angles; %inv(Tatt) * att_dot_cmd;

== matlab function gnc/INDI/Attitude/Pseudo-control/Limit_angles ==
  data: params input Bus: gnc_parameterBus; att_c input; ltd output single size=5; roll_limit input
function ltd = fcn(params,att_c,roll_limit)
ltd = zeros(5,1,'single');
alThBetPhi_prot = false(4,1);

alpha_max = params.limit.alpha_max*pi/180;
theta_max = params.limit.theta_max*pi/180;
beta_max = params.limit.beta_max*pi/180;

if att_c(1)>alpha_max
    ltd(1)=alpha_max;
    alThBetPhi_prot(1)=true;
else
    ltd(1) = att_c(1);
end

if att_c(2)>theta_max
    ltd(2)=theta_max;
    alThBetPhi_prot(2)=true;
else
    ltd(2) = att_c(2);
end

if att_c(3)>beta_max
    ltd(3)=beta_max;
    alThBetPhi_prot(3)=true;
elseif att_c(3)<-beta_max
    ltd(3)=-beta_max;
    alThBetPhi_prot(3)=true;
else
    ltd(3) = att_c(3);
end

ltd(4) = atan2(sin(att_c(4)),cos(att_c(4))); %limit psi between -pi and pi

if att_c(5)>roll_limit
    ltd(5)=roll_limit;
    alThBetPhi_prot(4)=true;
elseif att_c(5)<-roll_limit
    ltd(5)=-roll_limit;
    alThBetPhi_prot(4)=true;
else
    ltd(5) = att_c(5);
end

== matlab function gnc/Modal/scale_thr ==
  data: in input single; out output single
function out = fcn(in)

out = in;

out(4) = (in(4)+1)/2; %scale RC thrust from [-1,1] to [0,1]

== matlab function gnc/Mixer/scale_RC_thr ==
  data: in input single; out output single
function out = fcn(in)

out = in;
out(4) = 2*in(4)-1; %scale RC thrust from [0,1] to [-1,1]

== matlab function gnc/Modal/MATLAB Function ==
  data: ele_thr input size=2; axis_modes input; ele_thr_cmd output size=2
function ele_thr_cmd = fcn(ele_thr,axis_modes)


if axis_modes(4) <= 0 %direct thrust
    ele_thr_cmd = [ele_thr(1);single(0)];
else
    ele_thr_cmd = ele_thr;
end

== matlab function gnc/Modal/Command value selector ==
  data: k_vec input; chiError input; rc_mode input uint8; rollLimit input; psiCmd input; phi_dir input; C_ctrlLat output single; latCmd output single; C_ctrlLon output single size=[2,4]; Vcmd input; thetaCmd input; gammaCmd input; longCmd output single
function [C_ctrlLat,latCmd,C_ctrlLon,longCmd] = cmdSelector(k_vec,chiError,rc_mode,rollLimit,psiCmd,phi_dir,Vcmd,thetaCmd,gammaCmd)

longCmd     = single(zeros(4,1));
latCmd      = single(zeros(4,1));
C_ctrlLat	= single(zeros(2,4));
C_ctrlLon	= single(zeros(2,4));

kLat = k_vec(1);

% phi_cmd from chi
phi_cmd = chiError*kLat*max(Vcmd,10);
phi_ltd = min(rollLimit,max(-rollLimit,phi_cmd));

if rc_mode == uint8(1) %Test_control: theta, V in lon and phi, psi in lat
    %lon
    longCmd(1,1) = thetaCmd;
    longCmd(3,1) = Vcmd;
    C_ctrlLon(1,3)	= 1;
    C_ctrlLon(2,1)	= 1;
    
    %lat
    latCmd(3,1) = phi_dir;
    latCmd(4,1) = psiCmd;
    C_ctrlLat(1,3)	= 1; %phi
    C_ctrlLat(2,4)	= 1; %psi
elseif rc_mode == uint8(2) %Steady_state: gamma, V in lon and phi (direct), beta in lat
    %lon
    longCmd(3,1) = Vcmd;
    longCmd(4,1) = gammaCmd;
    C_ctrlLon(1,3)	= 1;
    C_ctrlLon(2,4)	= 1;
    
    %lat
    latCmd(3,1) = phi_dir;
    C_ctrlLat(1,3)	= 1; %phi
    C_ctrlLat(2,4)	= 1; %beta
else %Cruise control: gamma, V in lon and phi (from chi), beta in lat
    %lon
    longCmd(3,1) = Vcmd;
    longCmd(4,1) = gammaCmd;
    C_ctrlLon(1,3)	= 1;
    C_ctrlLon(2,4)	= 1;
    
    %lat
    latCmd(3,1) = phi_ltd;
    C_ctrlLat(1,3)	= 1; %phi
    C_ctrlLat(2,4)	= 1; %beta
end

== matlab function gnc/Subsystem1/MATLAB Function ==
  data: array_in input; array_out output
function array_out = fcn(array_in)

array_out = single(zeros(1,size(array_in,1)*size(array_in, 2)));

for i = 1:size(array_in,1)
    for j = 1:size(array_in,2)
        array_out(i+(size(array_in,1))*(j-1)) = array_in(i,j);
    end
end

== matlab function gnc/Modal/Gains2 ==
  data: KI_lat output; KP_lat output; KI_lon output; parameters input; KP_lon output; KP_turn output; KG_lat output
function [KI_lat, KP_lat, KI_lon, KP_lon, KP_turn, KG_lat] = generate_gain_matrices(parameters)

KP_lon = zeros(2,4,'single');
KI_lon = zeros(2,2,'single');
KP_lat = zeros(2,4,'single');
KI_lat = zeros(2,2,'single');
KG_lat = zeros(2,1,'single');

KP_lon(1,1) = parameters.lonCruise.K_ALPHA_ETA;
KP_lon(1,2) = parameters.lonCruise.K_Q_ETA;
KP_lon(1,3) = parameters.lonCruise.K_V_ETA;
KP_lon(1,4) = parameters.lonCruise.K_GAMMA_ETA;
KP_lon(2,1) = parameters.lonCruise.K_ALPHA_DELTA;
KP_lon(2,2) = parameters.lonCruise.K_Q_DELTA;
KP_lon(2,3) = parameters.lonCruise.K_V_DELTA;
KP_lon(2,4) = parameters.lonCruise.K_GAMMA_DELTA;
KI_lon(1,1) = parameters.lonCruise.I_V_ETA;
KI_lon(1,2) = parameters.lonCruise.I_GAMMA_ETA;
KI_lon(2,1) = parameters.lonCruise.I_V_DELTA;
KI_lon(2,2) = parameters.lonCruise.I_GAMMA_DELTA;
KP_lat(1,1) = parameters.latCruise.K_R_XI;
KP_lat(1,2) = parameters.latCruise.K_P_XI;
KP_lat(1,3) = parameters.latCruise.K_PHI_XI;
KP_lat(1,4) = parameters.latCruise.K_BETA_XI;
KP_lat(2,1) = parameters.latCruise.K_R_ZETA;
KP_lat(2,2) = parameters.latCruise.K_P_ZETA;
KP_lat(2,3) = parameters.latCruise.K_PHI_ZETA;
KP_lat(2,4) = parameters.latCruise.K_BETA_ZETA;
KI_lat(1,1) = parameters.latCruise.I_PHI_XI;
KI_lat(1,2) = parameters.latCruise.I_BETA_XI;
KI_lat(2,1) = parameters.latCruise.I_PHI_ZETA;
KI_lat(2,2) = parameters.latCruise.I_BETA_ZETA;
KP_turn     = parameters.lonCruise.K_TURN;
KG_lat(1)   = parameters.latCruise.P_CHI;

== matlab function gnc/Modal/Subsystem2/MATLAB Function ==
  data: x input; trigger output; x0 output; external input; u0 input; u input size=1; param input
function [trigger, x0] = fcn(x,external, u0, u,param)

limits = param.lonCruise.mainGain*[-1,1];

u_ltd = bound(u,limits);
x0 = bound(u0-u_ltd,limits-u_ltd);

trigger = false;
if external
    trigger = true;
else
    if u+x > limits(2)
        trigger = true;
        x0 = limits(2)-u;
    elseif u+x < limits(1)
        trigger = true;
        x0 = limits(1)-u;
    end
end
%x0 = bound(x0,limits);%% test!!!
end

function x_ltd = bound(x,limits)
x_ltd = max(min(x,limits(2)),limits(1));
end

== matlab function gnc/INDI/Path/Incremental_inversion/Attitude_Command_Generator ==
  data: gachiv_dot_e input size=3; abmu_m input size=3; params input Bus: gnc_parameterBus; gav_m input; q_dyn input; gncConsts parameter; att_inc_reciprocal output size=3; att_inc_inversion output size=3
function [att_inc_reciprocal,att_inc_inversion]= track_control(gachiv_dot_e,abmu_m,params,gav_m,q_dyn,gncConsts)
%% Parameters
m        = gncConsts.vehicle_m;
g        = gncConsts.g;
S        = gncConsts.vehicle_S;
Va_min   = single(5);
V_air    = max(Va_min,gav_m(2));
AR       = (gncConsts.vehicle_b)^2/S;
k        = 1/(pi*AR*params.indi.oswald);
Cl_alpha = 2*pi*AR/(AR+2);
Cd_alpha = 2*k*(Cl_alpha)^2*abmu_m(1);
thr_coeff= g*params.indi.EFF_DELTA/2; % T_delta: mapping thrust lever in [-1,1] -> thrust force

%% Full B matrix inversion
% [ dgam/dalp  dgam/dmu dgam/ddel  dgam/dbet  ]
% [ dchi/dalp  dchi/dmu dchi/ddel  dchi/dbet  ]
% [ dV/dalp    dV/dmu   dV/ddel    dV/dbet    ]
B = 1/(V_air*m)*[Cl_alpha*cos(abmu_m(3))*q_dyn*S,tan(abmu_m(3))*cos(gav_m(1))*m*g,thr_coeff*cos(abmu_m(3))*sin(abmu_m(1));
                (Cl_alpha*sin(abmu_m(3))*q_dyn*S)/cos(gav_m(1)),m*g,(thr_coeff*sin(abmu_m(3))*sin(abmu_m(1)))/cos(gav_m(1));
                V_air*Cd_alpha*q_dyn*S,0,V_air*thr_coeff*cos(abmu_m(1))];

att_inc_inversion = B(:,1:3)\gachiv_dot_e; %alpha_inc, mu_inc, thr_inc

%% Reciprocals of selected B elements -> SISO
B_rec = [diag([1/B(1,1),1/B(2,2),1/B(3,3)])]; % diag([dalp/dgam, dmu/dchi, ddel/dV],dbet/dV)
att_inc_reciprocal = B_rec*gachiv_dot_e; %alpha_inc, mu_inc, thr_inc
    
end

== matlab function gnc/INDI/MATLAB Function2 ==
  data: act_m input; act_limit input; inc_margins output size=[3,2]
function inc_margins = fcn(act_m,act_limit)

%% Limit actuator increments to maximum actuator deflection angles
upper_bounds = act_limit*pi/180; %[xi_max;eta_max;zeta_max]
lower_bounds = -upper_bounds;

inc_margins = [lower_bounds-act_m(1:3),upper_bounds-act_m(1:3)];

== matlab function gnc/Guidance/Envelope Protection ==
  data: param input Bus: gnc_parameterBus; cmd_out output Bus: guidance_cmd; cmd_in input Bus: guidance_cmd
function cmd_out  = fcn(param,cmd_in)

cmd_out = cmd_in;

if cmd_in.trk_cmd(1) < param.limit.gammaMin/180*pi %FPA too low
    cmd_out.trk_cmd(1) = param.limit.gammaMin/180*pi;
elseif cmd_in.trk_cmd(1) > param.limit.gammaMax/180*pi %FPA too high
    cmd_out.trk_cmd(1) = param.limit.gammaMax/180*pi;
end

if cmd_in.trk_cmd(3) < param.limit.vel_min %velocity too small during FLT phase
    cmd_out.trk_cmd(3) = param.limit.vel_min;
elseif cmd_in.trk_cmd(3) > param.limit.vel_max
    cmd_out.trk_cmd(3) = param.limit.vel_max;
end

== matlab function gnc/INDI/Path/MATLAB Function ==
  data: acc_k input; Vk input; gachi_dot output single size=2; v_dot output single size=1
function [gachi_dot,v_dot] = fcn(acc_k,Vk)
if Vk < single(0.5)
    Vk = single(0.5);
end

gachi_dot = [-acc_k(3);acc_k(2)]/Vk;
v_dot = acc_k(1);

== matlab function gnc/Modal/Subsystem2/MATLAB Function1 ==
  data: x input; trigger output; x0 output; external input; u0 input; u input; param input
function [trigger, x0] = fcn(x,external, u0, u,param)

limits = param.lonCruise.mainGain*[-1,1];

x0 = bound(u0-u,limits-u);

trigger = false;
if external
    trigger = true;
else
    if u+x > limits(2)
        trigger = true;
        x0 = limits(2)-u;
    elseif u+x < limits(1)
        trigger = true;
        x0 = limits(1)-u;
    end
end
x0 = bound(x0,limits);%% test!!!
end

function x_ltd = bound(x,limits)
x_ltd = max(min(x,limits(2)),limits(1));
end

== matlab function gnc/Modal/lateral ctrl1 ==
  data: k_turn input; phi input; u0 output
function u0 = turnComp(k_turn,phi)
phi = min(max(phi,-pi/3),pi/3);
u0  = [k_turn*(1/cos(phi)-cos(phi)); 0]; % Turn Compensation

== matlab function gnc/INDI/Path/Pseudo-control/MATLAB Function2 ==
  data: phi input; gamma_dot_ffw output single
function gamma_dot_ffw = turn_comp(phi)

gamma_dot_ffw=single(0);

%if params.indi.turn_comp
%    gamma_dot_ffw=single(0);
%end

== matlab function gnc/INDI/Path/Pseudo-control/Original/MATLAB Function1 ==
  data: u input; y output single
function y = angle_sat(u)

y = u;
if u(2) > single(pi)
    y(2) = u(2) - single(2*pi);
elseif u(2) < -single(pi)
    y(2) = u(2) + single(2*pi);
end

end

== matlab function gnc/INDI/Path/Pseudo-control/Original/MATLAB Function2 ==
  data: phi input; gamma_dot_ffw output single
function gamma_dot_ffw = turn_comp(phi)

gamma_dot_ffw=single(0);

%if params.indi.turn_comp
%    gamma_dot_ffw=single(0);
%end

== matlab function gnc/MATLAB Function2 ==
  data: params input; controls output; indi input; modal input
function controls = fcn(params, indi, modal)

if params.controller_selector == 1
    controls = modal;
else
    controls = indi;
end

== matlab function gnc/INDI/Rates to surfaces&brakes/Diff and Filter IMU/MATLAB Function ==
  data: omega input; num output; den output; zeta input
function [num,den] = fcn(omega,zeta)
w = omega*2*pi; %rad/s
z = zeta;
T = single(0.01);

scale = T^2*w^2+4*T*w*z+4;

%Tustin approximation of second order lowpass with derivative
% diff_num = [2*T*w^2 0 -2*T*w^2]/scale;
% diff_den = [T^2*w^2+4*T*w*z+4 2*T^2*w^2-8 T^2*w^2-4*T*w*z+4]/scale;

%Tustin approximation of second order lowpass
num = [T^2*w^2, 2*T^2*w^2, T^2*w^2]/scale;
den = [T^2*w^2+4*T*w*z+4 2*T^2*w^2-8 T^2*w^2-4*T*w*z+4]/scale;

== matlab function gnc/Guidance/Cruise_Guidance ==
  settings: updateMethod=DISCRETE
  data: commands output single; curr_wp output size=4; pos input single; params input Bus: gnc_parameterBus; wp_count input single; Va input; waypoints input single size=[3,20]; resetWP input; wps output single size=[3,20]
function [commands,curr_wp,wps] = Cruise_Guidance(pos,params,wp_count,Va,waypoints,resetWP)
persistent CurrentWP_ID PreviousWP_ID

assert (wp_count <= 10000)
wps = zeros(3,20,'single');

%% Assign constants
if wp_count == single(0) || wp_count > single(20)
    WayPoints = zeros(3,20,'single');
else
    WayPoints = waypoints;
end

if (isempty(CurrentWP_ID) || resetWP)
    CurrentWP_ID = single(1);
    PreviousWP_ID   = single(20);
end

%% Instantiate output
curr_wp = [CurrentWP_ID;WayPoints(:,CurrentWP_ID)];

%% Set local variables
K_H = params.guidance.K_H;
K_V = params.guidance.K_V;
if pos(3)>-40 %AGL within 40m
    rollLim = min(single(40*pi/180),params.limit.phi_max); %prevent lidar orientation_invalid
else
    rollLim = min(single(45*pi/180),params.limit.phi_max);
end
%

%% Scitech
if params.h_loiter == 0
    h_loiter = -50-params.h_fake; %down positive
else
    h_loiter = -params.h_loiter; %down positive
end

%% Controller methods
Vcmd = params.guidance.v_cmd;
%Use all waypoints for cruise tracking
wps_act = [WayPoints(1:2,1:wp_count);min(h_loiter*ones(1,wp_count),WayPoints(3,1:wp_count))];
wp_num = single(size(wps_act,2));
wps(:,1:wp_num) = wps_act;

[gammaCmd,chiCmd,CurrentWP_ID,PreviousWP_ID] = path_tracking(pos,Va,wps,rollLim,CurrentWP_ID,PreviousWP_ID,K_H,K_V,wp_num);

% Summarize command values
commands = [gammaCmd, chiCmd, Vcmd]';

end

function [gamma_cmd, chi_cmd, wp_curr_id, wp_prev_id] = path_tracking(pos, Vk, wp, rollLim, wp_curr_id, wp_prev_id, k_h, k_v, wp_count)
[gamma_cmd, chi_cmd] = path_controller(pos,Vk,wp(:,wp_curr_id),wp(:,wp_prev_id),k_h,k_v);
[wp_curr_id,wp_prev_id] = wpSwitching(pos,Vk,wp,rollLim,wp_curr_id,wp_prev_id,wp_count); %Check the switching conditions
if wp_count>0 && wp_curr_id > wp_count
    wp_curr_id = wp_count;
end
end

function [gamma_cmd, chi_cmd] = path_controller(r, Vk, currWP, prevWP, k_h, k_v)
% Inputs:
%   - r          The current position of the Aircraft -> [North, East, Down]
%   - Vk         Ground Speed of the Aircraft
%   - WP         A matrix containing all WayPoints (one Waypoint(WP) per column: [North, East, Down]')
%   - curr_WP_id The ID/row number of the current WP
%   - prevWP     The last WP [North, East, Down]'
%
% Outputs:
%   - gamma_cmd  The commanded flight-path angle
%   - chi_cmd    The commanded pitch angle

ky =  0.895413552164936/4*k_h;
kz =  1.9893916106768/4*k_v;
maxClimb   = 10;
maxDescent = 10;
% gammaMax   = 8/180*pi;

dr = (currWP-prevWP);
gamma0 = atan2(-dr(3),norm(dr(1:2)));
chi0   = atan2(dr(2),dr(1));

TrE = [cos(gamma0)*cos(chi0) cos(gamma0)*sin(chi0) -sin(gamma0);...
    -sin(chi0) cos(chi0) 0;...
    sin(gamma0)*cos(chi0) sin(gamma0)*sin(chi0) cos(gamma0)];

rrFZ = TrE*(r-prevWP);

% Pseudo Control
uL = - ky * rrFZ(2);
uV = - kz * rrFZ(3);

% Lateral Inversion
Vk = max(Vk,max(maxClimb,maxDescent));
if uL > Vk*cos(gamma0)
    chi_cmd = pi/2 + chi0;
elseif uL < - Vk*cos(gamma0)
    chi_cmd = -pi/2 + chi0;
else
    asin_limiterLat = uL/(Vk*cos(gamma0));
    asin_limiterLat = min(max(asin_limiterLat,-1),1);
    chi_cmd = asin(asin_limiterLat) + chi0;
end

% Vertical Inversion
a = -cos(gamma0);
b = sin(gamma0)*cos(chi_cmd - chi0);

uVmax = Vk*sqrt(a^2+b^2);
if uV > uVmax
    gamma_cmd = -pi/2+atan2(b,-a);
elseif uV < -uVmax
    gamma_cmd = pi/2+atan2(b,-a);
else
    c = uV / Vk;
    asin_limiterLon = c/sqrt(a^2+b^2);
    asin_limiterLon = min(max(asin_limiterLon,-1),1);
    gamma_cmd = -asin(asin_limiterLon)+atan2(b,-a);
end

% gammaMin  = max(-asin(maxDescent/Vk),-gammaMax);
% gammaMax  = min(asin(maxClimb/Vk),gammaMax);
% gamma_cmd = min(max(gamma_cmd,gammaMin),gammaMax);
end

function [currWP_id, prevWP_id] = wpSwitching(r, Vk, wp, rollLim, currWP_id, prevWP_id, wp_count)
% Inputs:
%   - r         The current position of the Aircraft -> [North, East, Down]
%   - Vk        Ground Speed of the Aircraft
%   - wp        A matrix containing all WayPoints (one Waypoint(WP) per column: [North, East, Down]')
%   - currWP_id The ID/row number of the current WP
%   - prevWP    The last WP [North, East, Down]'
%
% Outputs:
%   - currWP_id The ID/row number of the current WP - Must only be changed if the switch condition is fullfilled
%   - prevWP    The last WP [North, East, Down] - Must only be changed if the switch condition is fullfilled
if currWP_id + 1 > wp_count
    nextWP_id = single(1);
else
    nextWP_id = currWP_id + single(1);
end
PreviousWP = wp(:,prevWP_id);
CurrentWP = wp(:,currWP_id);
NextWP    = wp(:,nextWP_id);

cPath  = (CurrentWP-PreviousWP);
gamma0 = atan2(-cPath(3),norm(cPath(1:2)));
chi0   = atan2(cPath(2),cPath(1));

TrE = [cos(gamma0)*cos(chi0) cos(gamma0)*sin(chi0) -sin(gamma0);...
    -sin(chi0) cos(chi0) 0;...
    sin(gamma0)*cos(chi0) sin(gamma0)*sin(chi0) cos(gamma0)];
rrFZ   = TrE*(r-PreviousWP);

nPath = NextWP - CurrentWP;

acos_limiter = cPath'*nPath / (norm(cPath)*norm(nPath));
%disp(acos_limiter);
acos_limiter = min(max(acos_limiter,-1),1);
switchAngle = acos(acos_limiter);

if switchAngle >= single(150*pi/180)
    switchAngle = single(150*pi/180);
elseif switchAngle <= single(20*pi/180)
    switchAngle = single(20*pi/180);
end

turnRadius = Vk^2 / (tan(rollLim)*9.81);
switchRadius = turnRadius*tan(switchAngle/2);

if (norm(cPath) - rrFZ(1) < switchRadius)
    prevWP_id = currWP_id;
    currWP_id = nextWP_id;
end
end

== matlab function gnc/INDI/Rates to surfaces&brakes/Incremental_inversion/MATLAB Function3 ==
  data: ctrl_eff_inv output; J output; b_c_inv output; S output; param input; gncConsts parameter
function [ctrl_eff_inv,J,b_c_inv,S] = tbv(param,gncConsts)
b = gncConsts.vehicle_b;
chord=gncConsts.vehicle_c;
S=gncConsts.vehicle_S;

b_c_inv=[1/b 0 0 ; 0 1/chord 0 ;0 0 1/b];

Jxx = param.indi.inertia_xx;
Jxy = param.indi.inertia_xy;
Jyy = param.indi.inertia_yy;
Jyz = param.indi.inertia_yz;
Jzz = param.indi.inertia_zz;
Jxz = param.indi.inertia_xz;
J = [Jxx Jxy Jxz;Jxy Jyy Jyz;Jxz Jyz Jzz];

Cmele  = param.indi.EFF_ETA_M; 
Clail  = param.indi.EFF_XI_L;
Cnail  = param.indi.EFF_XI_N;
Clrud  = param.indi.EFF_ZETA_L;
Cnrud  = param.indi.EFF_ZETA_N;
ctrl_eff_inv = 1/(Clail*Cnrud - Clrud*Cnail)*[Cnrud 0 -Clrud; 0 (Clail*Cnrud - Clrud*Cnail)/Cmele 0; -Cnail 0 Clail]; % matrix of aerodynamic coefficients

== matlab function gnc/Modal/limit chi error ==
  data: u input; y output single
function y = angle_sat(u)

if u > pi
    y = u - single(2*pi);
elseif u < -pi
    y = u + single(2*pi);
else
    y = u;
end

end
